simulink model "Modello_Completo"  (R2019a)
settings: Solver=VariableStepAuto  StartTime=0.0  StopTime=50000  RelTol=1e-3
values from neighbouring files (symbols this model uses):
  A = [-5.61e-05 0 0 0 0 0 0 1 1 6.793e-05 -0.00137658 -0.00155076 ... (81 elements, 9x9)]    [wrokspace_definitivo.mat]
  B = [5.61e-05 0 0 0 0 0 0 0 0 0 0.0004421 0 ... (45 elements, 9x5)]    [wrokspace_definitivo.mat]
  C = [1 0 0 0 0 0 0 0 0 0 1 0 ... (81 elements, 9x9)]    [wrokspace_definitivo.mat]
  D = [0 0 0 0 0 0 0 0 0 0 0 0 ... (45 elements, 9x5)]    [wrokspace_definitivo.mat]
undefined symbols (not defined in the file or in its folder): amplifier2, amplifier3, exciter2, exciter3, PID_new_2, PID_new_3
settings Model: Creator=leonardo  LastModifiedBy=leonardo
settings DataIOCC: ReturnWorkspaceOutputs=off
settings DebuggingCC: ArithmeticOperatorsInVariantConditions=warning

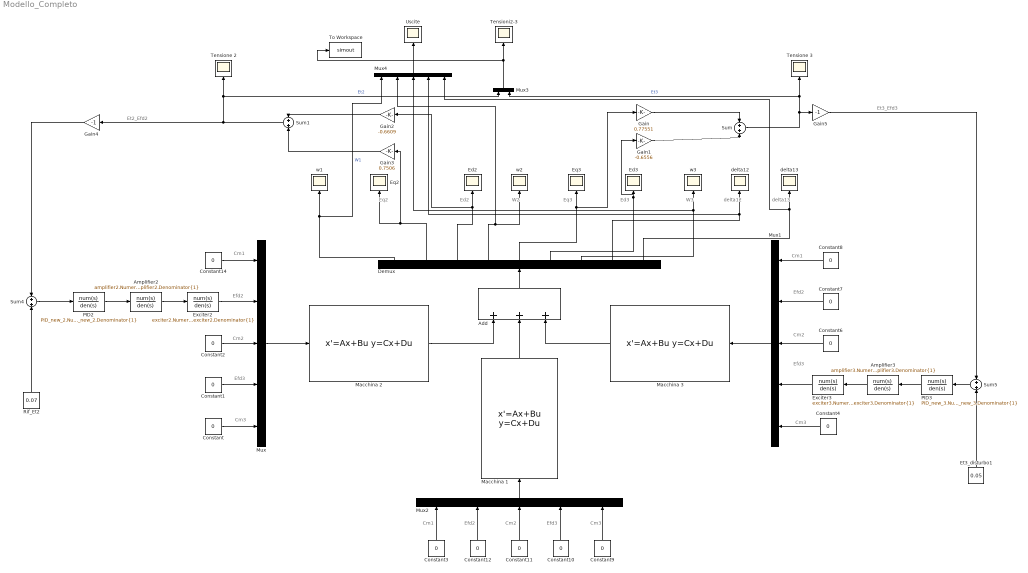
== system Modello_Completo ==
  note: Cm3
  note: Efd3
  note: Cm2
  note: Efd2
  note: Cm1
  note: Et2_Efd2
  note: Et3_Efd3
  note: delta13
  note: delta12
  note: W3
  note: Ed3
  note: Eq3
  note: W2
  note: Ed2
  note: Eq2
  note: Cm1
  note: Efd2
  note: Cm2
  note: Efd3
  note: Cm3
  note: Cm1
  note: Efd2
  note: Cm2
  note: Cm3
  note: Efd3
  Add : Sum  Inputs=+++
  Amplifier2 : TransferFcn  Numerator=amplifier2.Numerator{1}  Denominator=amplifier2.Denominator{1}
  Amplifier3 : TransferFcn  Numerator=amplifier3.Numerator{1}  Denominator=amplifier3.Denominator{1}
  Constant{,1..4,6..12,14} (13 alike) : Constant  Value=0
  Demux : Demux  Outputs=9
  Ed2 : Scope
  Ed3 : Scope
  Eq2 : Scope
  Eq3 : Scope
  Et3_disturbo1 : Constant  Value=0.05
  Exciter2 : TransferFcn  Numerator=exciter2.Numerator{1}  Denominator=exciter2.Denominator{1}
  Exciter3 : TransferFcn  Numerator=exciter3.Numerator{1}  Denominator=exciter3.Denominator{1}
  Gain : Gain  Gain=0.77551
  Gain1 : Gain  Gain=-0.6556
  Gain2 : Gain  Gain=-0.6609
  Gain3 : Gain  Gain=0.7506
  Gain4 : Gain  Gain=-1
  Gain5 : Gain  Gain=-1
  Macchina 1 : StateSpace  A=A  B=B  C=C  D=D  InitialCondition=0
  Macchina 2 : StateSpace  A=A  B=B  C=C  D=D  InitialCondition=[0 0 0 0 0 0 0 0 0]
  "Macchina 3 " : StateSpace  A=A  B=B  C=C  D=D  InitialCondition=[0 0 0 0 0 0 0 0 0]
  Mux{,1..2,4} (4 alike) : Mux  Inputs=5
  Mux3 : Mux  Inputs=2
  PID2 : TransferFcn  Numerator=PID_new_2.Numerator{1}  Denominator=PID_new_2.Denominator{1}
  PID3 : TransferFcn  Numerator=PID_new_3.Numerator{1}  Denominator=PID_new_3.Denominator{1}
  Rif_Et2 : Constant  Value=0.07
  Sum : Sum  Inputs=+|+
  Sum1 : Sum  Inputs=+|+
  Sum4 : Sum
  Sum5 : Sum
  Tensione 2 : Scope
  Tensione 3 : Scope
  Tensioni2-3 : Scope
  To Workspace : ToWorkspace  VariableName=simout  SaveFormat=Timeseries  SampleTime=0.5
  Uscite : Scope
  delta12 : Scope
  delta13 : Scope
  w1 : Scope
  w2 : Scope
  w3 : Scope
  wires:
  Constant/1 -> Mux/5
  Constant1/1 -> Mux/4
  Mux/1 -> Macchina 2/1
  Demux/2 -> Gain3/1, Eq2/1
  Demux/3 -> Gain2/1, Ed2/1
  Demux/5 -> Gain/1, Eq3/1
  Demux/6 -> Gain1/1, Ed3/1
  Demux/7 -> Mux4/3, w3/1
  Demux/8 -> Mux4/4, delta12/1
  Demux/9 -> Mux4/5, delta13/1
  Add/1 -> Demux/1
  Macchina 2/1 -> Add/1
  "Macchina 3 "/1 -> Add/3
  Macchina 1/1 -> Add/2
  Constant6/1 -> Mux1/3
  Constant7/1 -> Mux1/2
  Mux1/1 -> "Macchina 3 "/1
  Constant8/1 -> Mux1/1
  Constant10/1 -> Mux2/4
  Constant12/1 -> Mux2/2
  Constant11/1 -> Mux2/3
  Constant9/1 -> Mux2/5
  Mux2/1 -> Macchina 1/1
  Constant14/1 -> Mux/1
  Demux/1 -> Mux4/1, w1/1  "W1"
  Gain/1 -> Sum/1
  Gain1/1 -> Sum/2
  Sum/1 -> Gain5/1, Tensione 3/1, Mux3/2  "Et3"
  Gain3/1 -> Sum1/2
  Gain2/1 -> Sum1/1
  Sum1/1 -> Gain4/1, Mux3/1, Tensione 2/1  "Et2"
  PID3/1 -> Amplifier3/1
  Gain4/1 -> Sum4/1
  Gain5/1 -> Sum5/1
  Amplifier2/1 -> Exciter2/1
  Amplifier3/1 -> Exciter3/1
  Demux/4 -> Mux4/2, w2/1
  Constant2/1 -> Mux/3
  Constant4/1 -> Mux1/5
  Constant3/1 -> Mux2/1
  Sum4/1 -> PID2/1
  PID2/1 -> Amplifier2/1
  Sum5/1 -> PID3/1
  Mux3/1 -> To Workspace/1, Tensioni2-3/1
  Exciter3/1 -> Mux1/4
  Exciter2/1 -> Mux/2
  Mux4/1 -> Uscite/1
  Rif_Et2/1 -> Sum4/2
  Et3_disturbo1/1 -> Sum5/2
